simulink model "eq_analysis"  (R2013b)
settings: Solver=ode45  StartTime=0.0  StopTime=10.0  RelTol=1e-3
values from neighbouring files (symbols this model uses):
  Ac = [0 1;-wn(i)^2 -2*dmp(index)*wn(i)]    [hw8_plus.m]
  Bc = [0; -1]    [hw8_plus.m]
  Cc = [1 0;[-wn(i)^2 -2*dmp(index)*wn(i)]]    [hw8_plus.m]
  Dc = [0;0]    [hw8_plus.m]
  dt = tt_acc(2,1)-tt_acc(1,1)    [hw8_plus.m]
settings Model: Creator=chang  LastModifiedBy=chang

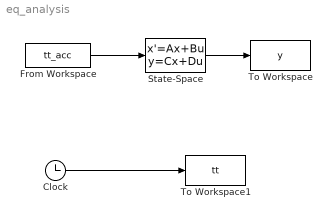
== system eq_analysis ==
  Clock : Clock
  From Workspace : FromWorkspace  VariableName=tt_acc  SampleTime=dt  OutputAfterFinalValue=Setting to zero
  State-Space : StateSpace  A=Ac  B=Bc  C=Cc  D=Dc  X0=0
  To Workspace : ToWorkspace  VariableName=y  SampleTime=-1
  To Workspace1 : ToWorkspace  VariableName=tt  SampleTime=-1
  wires:
  From Workspace/1 -> State-Space/1
  State-Space/1 -> To Workspace/1
  Clock/1 -> To Workspace1/1
